simulink library "determineSimulationPhase_ul"  (R2018a)
settings: Solver=VariableStepAuto  StartTime=0.0  StopTime=10.0  RelTol=1e-3
undefined symbols (not defined in the file or in its folder): ctrl
libraries: simulink x1, resettableCounter x1
settings Model: Creator=mitch  LastModifiedBy=mitch

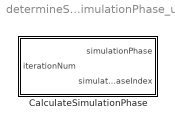
== system determineSimulationPhase_ul ==
  CalculateSimulationPhase : Subsystem

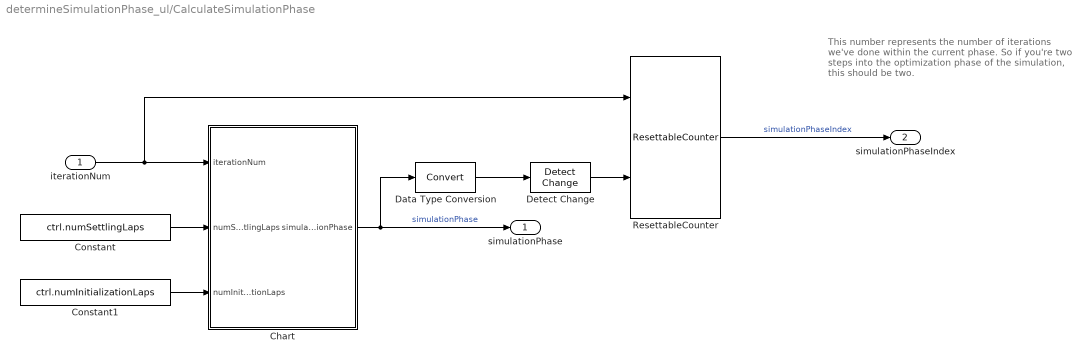
== system determineSimulationPhase_ul/CalculateSimulationPhase ==
  note: This number represents the number of iterations
      |  we've done within the current phase.  So if you're
      | two steps into the optimization phase of the
      | simulation, this should be two.
  iterationNum : Inport
  Chart : Stateflow chart  TreatAsAtomicUnit=on
  Constant : Constant  Value=ctrl.numSettlingLaps
  Constant1 : Constant  Value=ctrl.numInitializationLaps
  Data Type Conversion : DataTypeConversion
  Detect Change : simulink/Logic and Bit Operations/Detect Change  vinit=0  OutDataTypeStr=boolean
  ResettableCounter : resettableCounter/ResettableCounter
  simulationPhase : Outport  OutDataTypeStr=Enum: simulationPhase_enum
  simulationPhaseIndex : Outport  Port=2
  wires:
  Constant/1 -> Chart/2(numSettlingLaps)
  Constant1/1 -> Chart/3(numInitializationLaps)
  iterationNum/1 -> ResettableCounter/1, Chart/1(iterationNum)
  ResettableCounter/1 -> simulationPhaseIndex/1  "simulationPhaseIndex"
  Chart/1(simulationPhase) -> Data Type Conversion/1, simulationPhase/1  "simulationPhase"
  Detect Change/1 -> ResettableCounter/2
  Data Type Conversion/1 -> Detect Change/1

== stateflow chart determineSimulationPhase_ul/CalculateSimulationPhase/Chart ==
  state SETTLING
  state INITIALIZATION
  state OPTIMIZATION
  (default) -> SETTLING
  SETTLING -> INITIALIZATION : [iterationNum>numSettlingLaps]
  INITIALIZATION -> OPTIMIZATION : [iterationNum>numSettlingLaps+numInitializationLaps]
  data: iterationNum input; numSettlingLaps input; numInitializationLaps input; simulationPhase output Enum: simulationPhase_enum
